simulink model "EKFSim_R2016b"  (R2018b)
settings: Solver=VariableStepAuto  StartTime=0.0  StopTime=22500  RelTol=1e-3
undefined symbols (not defined in the file): sigbuilder_block
libraries: fl_lib x7, nesl_utility x7
settings Model: Creator=WL  LastModifiedBy=Alter
settings SFSimCC: SimUseLocalCustomCode=off
settings RTWCC: RTWUseLocalCustomCode=off
settings CodeAppCC: StateflowObjectComments=on

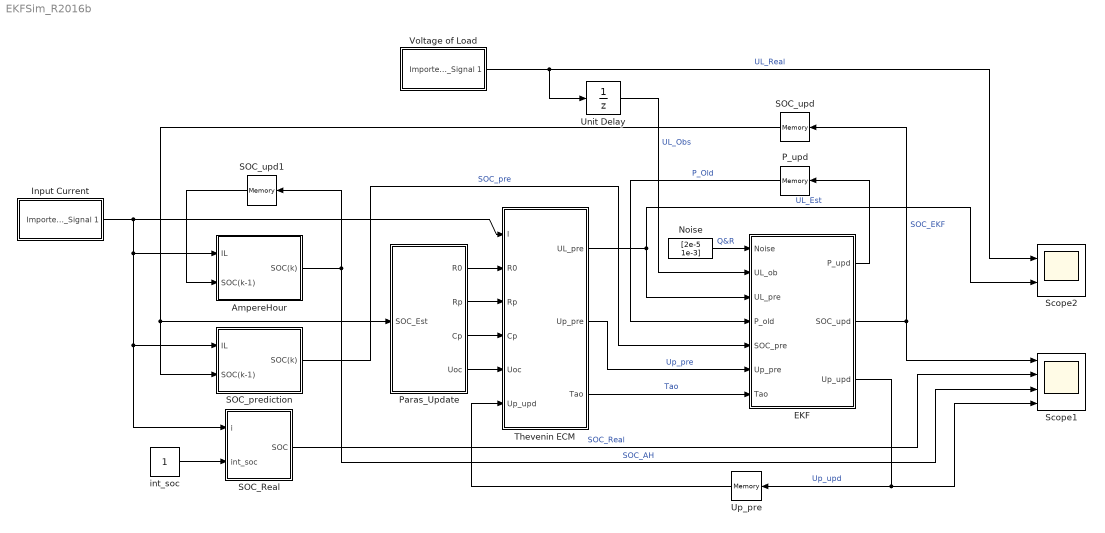
== system EKFSim_R2016b ==
  AmpereHour : Subsystem
  EKF : MATLAB Function  TreatAsAtomicUnit=on
  Input Current : Subsystem  Tag=STV Subsys  LoadFcn=sigbuilder_block('load');  StartFcn=sigbuilder_block('start');  StopFcn=sigbuilder_block('stop');  ClipboardFcn=sigbuilder_block('clipboard');  mask(Sigbuilder block){tuvar=[0:10]}
      mask help: Simulink:masks:SigbuilderBlock_MD
      mask init:
      | if ~strcmp(get_param(bdroot(gcbh),'SimulationStatus'),'stopped') tuvar = sigbuilder_block('maskInit'); end
      settings: CopyFcn=sigbuilder_block('copy');  DeleteFcn=sigbuilder_block('delete');  ModelCloseFcn=sigbuilder_block('modelClose');  PreSaveFcn=sigbuilder_block('preSave');  PauseFcn=sigbuilder_block('pause');  ContinueFcn=sigbuilder_block('continue');  NameChangeFcn=sigbuilder_block('namechange');  OpenFcn=sigbuilder_block('open',[6 51 1012.5 460.5 ]);  CloseFcn=sigbuilder_block('close');
      mask Display: plot(0, 0, 100, 100,[2, 2, 32, 32, 2], [68, 8, 8, 68, 68],[32, 2], [38, 38], [32, 19, 2],[53, 60, 44], [32, 17, 17, 2],[16, 16, 31, 31]);txt = getActiveGroup(gcbh);text(2, 100, txt,'verticalAlignment', 'top');
  Noise : Constant  Value=[2e-5 1e-3]
  P_upd : Memory  InitialCondition=[0.02 0 0 0.01]  InheritSampleTime=on  LinearizeAsDelay=on
  Paras_Update : Subsystem
  SOC_Real : Subsystem
  SOC_prediction : Subsystem
  SOC_upd : Memory  InitialCondition=1  InheritSampleTime=on  LinearizeAsDelay=on
  SOC_upd1 : Memory  InitialCondition=1  InheritSampleTime=on  LinearizeAsDelay=on
  Scope1 : Scope  NumInputPorts=4
  Scope2 : Scope  NumInputPorts=2
  Thevenin ECM : Subsystem
  Unit Delay : UnitDelay  InitialCondition=4.107  SampleTime=0.1
  Up_pre : Memory  InheritSampleTime=on  LinearizeAsDelay=on
  Voltage of Load : Subsystem  Tag=STV Subsys  LoadFcn=sigbuilder_block('load');  StartFcn=sigbuilder_block('start');  StopFcn=sigbuilder_block('stop');  ClipboardFcn=sigbuilder_block('clipboard');  mask(Sigbuilder block){tuvar=[0:10]}
      mask help: Simulink:masks:SigbuilderBlock_MD
      mask init:
      | if ~strcmp(get_param(bdroot(gcbh),'SimulationStatus'),'stopped') tuvar = sigbuilder_block('maskInit'); end
      settings: CopyFcn=sigbuilder_block('copy');  DeleteFcn=sigbuilder_block('delete');  ModelCloseFcn=sigbuilder_block('modelClose');  PreSaveFcn=sigbuilder_block('preSave');  PauseFcn=sigbuilder_block('pause');  ContinueFcn=sigbuilder_block('continue');  NameChangeFcn=sigbuilder_block('namechange');  OpenFcn=sigbuilder_block('open',[6 51 1012.5 460.5 ]);  CloseFcn=sigbuilder_block('close');
      mask Display: plot(0, 0, 100, 100,[2, 2, 32, 32, 2], [68, 8, 8, 68, 68],[32, 2], [38, 38], [32, 19, 2],[53, 60, 44], [32, 17, 17, 2],[16, 16, 31, 31]);txt = getActiveGroup(gcbh);text(2, 100, txt,'verticalAlignment', 'top');
  int_soc : Constant
  wires:
  Paras_Update/4(Uoc) -> Thevenin ECM/5(Uoc)
  Paras_Update/1(R0) -> Thevenin ECM/2(R0)
  int_soc/1 -> SOC_Real/2(int_soc)
  Paras_Update/3(Cp) -> Thevenin ECM/4(Cp)
  Paras_Update/2(Rp) -> Thevenin ECM/3(Rp)
  Thevenin ECM/1(UL_pre) -> Scope2/2, EKF/3(UL_pre)  "UL_Est"
  Voltage of Load/1(Imported_Signal 1) -> Unit Delay/1, Scope2/1  "UL_Real"
  SOC_Real/1(SOC) -> Scope1/2  "SOC_Real"
  Thevenin ECM/2(Up_pre) -> EKF/6(Up_pre)  "Up_pre"
  Noise/1 -> EKF/1(Noise)  "Q&R"
  SOC_prediction/1(SOC(k)) -> EKF/5(SOC_pre)  "SOC_pre"
  P_upd/1 -> EKF/4(P_old)  "P_Old"
  SOC_upd/1 -> SOC_prediction/2(SOC(k-1)), Paras_Update/1(SOC_Est)
  EKF/1(P_upd) -> P_upd/1
  Thevenin ECM/3(Tao) -> EKF/7(Tao)  "Tao"
  EKF/3(Up_upd) -> Scope1/4, Up_pre/1  "Up_upd"
  Up_pre/1 -> Thevenin ECM/6(Up_upd)
  EKF/2(SOC_upd) -> Scope1/1, SOC_upd/1  "SOC_EKF"
  Unit Delay/1 -> EKF/2(UL_ob)  "UL_Obs"
  AmpereHour/1(SOC(k)) -> Scope1/3, SOC_upd1/1  "SOC_AH"
  Input Current/1(Imported_Signal 1) -> SOC_prediction/1(IL), SOC_Real/1(i), AmpereHour/1(IL), Thevenin ECM/1(I)
  SOC_upd1/1 -> AmpereHour/2(SOC(k-1))

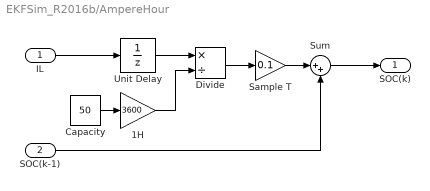
== system EKFSim_R2016b/AmpereHour ==
  IL : Inport
  SOC(k-1) : Inport  Port=2
  1H : Gain  Gain=3600
  Capacity : Constant  Value=50
  Divide : Product  Inputs=*/
  Sample T : Gain  Gain=0.1
  Sum : Sum  Inputs=|++
  Unit Delay : UnitDelay  SampleTime=0.15
  SOC(k) : Outport
  wires:
  Sample T/1 -> Sum/1
  Unit Delay/1 -> Divide/1
  SOC(k-1)/1 -> Sum/2
  IL/1 -> Unit Delay/1
  Sum/1 -> SOC(k)/1
  Capacity/1 -> 1H/1
  1H/1 -> Divide/2
  Divide/1 -> Sample T/1

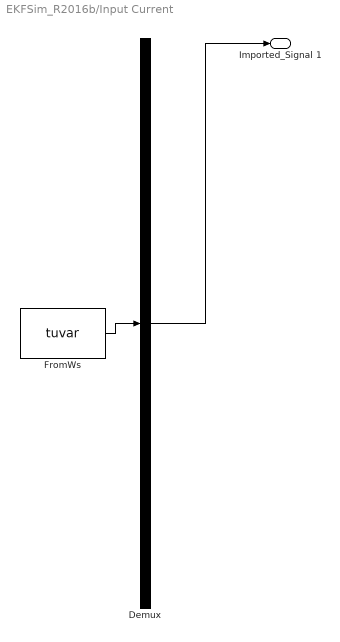
== system EKFSim_R2016b/Input Current ==
  Demux : Demux  Tag=STV Demux  Outputs=1
  FromWs : FromWorkspace  Tag=STV FromWs  VariableName=tuvar  SampleTime=0
      SigBuilderData=|
      | common.afterFinalStr = 'Extrapolate'
      | common.sampleTime = 0
      | dataSet.timeRange = [0 22502.2]
      | dataSet.name = 'I'
      | sbobj.Name = 'Signal Builder'
      | sbobj.Groups.Name = 'I'
      | sbobj.Groups.Signals.Name = 'Imported_Signal 1'
      | sbobj.Groups.Signals.XData = [0 0.05 0.1 0.15 0.2 0.25 0.3 0.35 0.4 0.45 0.5 0.55 ... (450045 elements, 1x450045)]
      | sbobj.Groups.Signals.YData = [0 0 0 0 0 0 0 0 0 0 0 0 ... (450045 elements, 1x450045)]
      | sbobj.Groups.TimeRange = [433.3 22935.5]
  Imported_Signal 1 : Outport
  wires:
  Demux/1 -> Imported_Signal 1/1
  FromWs/1 -> Demux/1

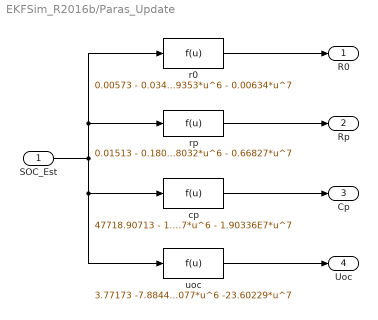
== system EKFSim_R2016b/Paras_Update ==
  SOC_Est : Inport
  cp : Fcn  Expr=47718.90713 - 1.00583E6*u^1 + 9.2653E6*u^2 - 3.91088E7*u^3 + 8.85892E7*u^4 - 1.11014E8*u^5 + 7.22811E7*u^6 - 1.90336E7*u^7
  r0 : Fcn  Expr=0.00573 - 0.03427*u^1 + 0.1455*u^2 - 0.32647*u^3 + 0.41465*u^4 - 0.28992*u^5 + 0.09353*u^6 - 0.00634*u^7
  rp : Fcn  Expr=0.01513 - 0.18008*u^1 + 1.05147*u^2 - 3.27616*u^3 + 5.79793*u^4 - 5.81819*u^5 + 3.08032*u^6 - 0.66827*u^7
  uoc : Fcn  Expr=3.77173 -7.88447*u^1 + 60.21383*u^2 -200.15462*u^3 + 345.34531*u^4 - 314.92282*u^5 + 141.34077*u^6 -23.60229*u^7
  R0 : Outport
  Rp : Outport  Port=2
  Cp : Outport  Port=3
  Uoc : Outport  Port=4
  wires:
  cp/1 -> Cp/1
  rp/1 -> Rp/1
  uoc/1 -> Uoc/1
  r0/1 -> R0/1
  SOC_Est/1 -> uoc/1, cp/1, rp/1, r0/1

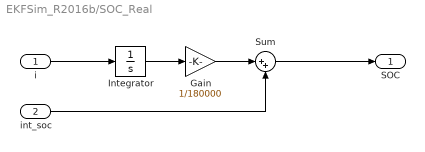
== system EKFSim_R2016b/SOC_Real ==
  i : Inport
  int_soc : Inport  Port=2
  Gain : Gain  Gain=1/180000
  Integrator : Integrator
  Sum : Sum  Inputs=|++
  SOC : Outport
  wires:
  Gain/1 -> Sum/1
  Integrator/1 -> Gain/1
  int_soc/1 -> Sum/2
  i/1 -> Integrator/1
  Sum/1 -> SOC/1

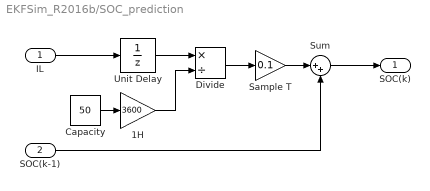
== system EKFSim_R2016b/SOC_prediction ==
  IL : Inport
  SOC(k-1) : Inport  Port=2
  1H : Gain  Gain=3600
  Capacity : Constant  Value=50
  Divide : Product  Inputs=*/
  Sample T : Gain  Gain=0.1
  Sum : Sum  Inputs=|++
  Unit Delay : UnitDelay  SampleTime=0.15
  SOC(k) : Outport
  wires:
  Sample T/1 -> Sum/1
  Unit Delay/1 -> Divide/1
  SOC(k-1)/1 -> Sum/2
  IL/1 -> Unit Delay/1
  Sum/1 -> SOC(k)/1
  Capacity/1 -> 1H/1
  1H/1 -> Divide/2
  Divide/1 -> Sample T/1

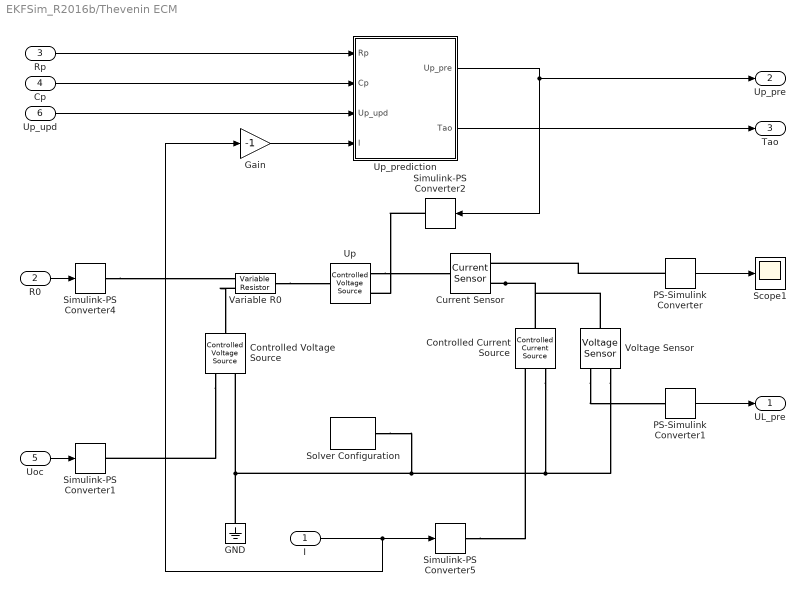
== system EKFSim_R2016b/Thevenin ECM ==
  I : Inport
  R0 : Inport  Port=2
  Rp : Inport  Port=3
  Cp : Inport  Port=4
  Uoc : Inport  Port=5
  Up_upd : Inport  Port=6
  Controlled Current Source : fl_lib/Electrical/Electrical Sources/Controlled Current Source
  Controlled Voltage Source : fl_lib/Electrical/Electrical Sources/Controlled Voltage Source
  Current Sensor : fl_lib/Electrical/Electrical Sensors/Current Sensor
  GND : fl_lib/Electrical/Electrical Elements/Electrical Reference
  Gain : Gain  Gain=-1
  PS-Simulink Converter : nesl_utility/PS-Simulink Converter  PhysicalDomain=network_engine_domain  SubClassName=ps_output  LeftPortType=input  RightPortType=output  PseudoPeriodic=off  Frequencies=[]  Unit=A  AffineConversion=off
  PS-Simulink Converter1 : nesl_utility/PS-Simulink Converter  PhysicalDomain=network_engine_domain  SubClassName=ps_output  LeftPortType=input  RightPortType=output  PseudoPeriodic=off  Frequencies=[]  Unit=V  AffineConversion=off
  Scope1 : Scope
  Simulink-PS Converter{1..2,4..5} (4 alike) : nesl_utility/Simulink-PS Converter  PhysicalDomain=network_engine_domain  SubClassName=ps_input  LeftPortType=input  RightPortType=output  PseudoPeriodic=off  Frequencies=[]  NoiseDistribution=none  NoiseParameters=[]  Unit=1  AffineConversion=off  FilteringAndDerivatives=zero  SimscapeFilterOrder=1  InputFilterTimeConstant=0.001  UdotUserProvided=0
  Solver Configuration : nesl_utility/Solver Configuration  PhysicalDomain=network_engine_domain  SubClassName=solver  LeftPortType=input  RightPortType=generic  Tones=[]  Harmonics=[]  SimulateNoise=off  Profile=off  UseLocalSampling=off  EnableSwitchedLinearOptims=on  FrequencyDomain=off  UseCCode=off  RelTol=0.001  AbsTol=1e-06  MinStep=1e-09  ToWorkspace=off  RevertToSquareIcSolve=off  NumHomotopyIterations=100  PhasorMode=off  PhasorModeNumHarmonics=1  DoDC=off  ResidualTolerance=1e-09  UseLocalSolver=off  LocalSolverChoice=NE_BACKWARD_EULER_ADVANCER  LocalSolverSampleTime=0.001  DoFixedCost=off  MaxNonlinIter=3  MaxModeIter=2  LinearAlgebra=Sparse  EquationFormulation=NE_TIME_EF  DelaysMemoryBudget=1024  AutomaticFiltering=on  FilteringTimeConstant=0.001  PartitionStorageMethod=AS_NEEDED  PartitionMemoryBudget=1024
  Up : fl_lib/Electrical/Electrical Sources/Controlled Voltage Source
  Up_prediction : MATLAB Function  TreatAsAtomicUnit=on
  Variable R0 : fl_lib/Electrical/Electrical Elements/Variable Resistor  Rmin=0 Ohm  i_specify=off  i_priority=None  i=0 A  i_nominal_specify=off  i_nominal_unit=A  i_nominal_value=1  v_specify=off  v_priority=None  v=0 V  v_nominal_specify=off  v_nominal_unit=V  v_nominal_value=1
  Voltage Sensor : fl_lib/Electrical/Electrical Sensors/Voltage Sensor
  UL_pre : Outport
  Up_pre : Outport  Port=2
  Tao : Outport  Port=3
  wires:
  PS-Simulink Converter1/1 -> UL_pre/1
  Uoc/1 -> Simulink-PS Converter1/1
  Cp/1 -> Up_prediction/2(Cp)
  Rp/1 -> Up_prediction/1(Rp)
  R0/1 -> Simulink-PS Converter4/1
  I/1 -> Gain/1, Simulink-PS Converter5/1
  PS-Simulink Converter/1 -> Scope1/1
  Up_prediction/1(Up_pre) -> Simulink-PS Converter2/1, Up_pre/1
  Up_upd/1 -> Up_prediction/3(Up_upd)
  Up_prediction/2(Tao) -> Tao/1
  Gain/1 -> Up_prediction/4(I)
  connections:
  Variable R0/LConn2 -- Controlled Voltage Source/LConn1
  Current Sensor/RConn2 -- Voltage Sensor/LConn1 -- Controlled Current Source/LConn1
  Voltage Sensor/RConn2 -- Controlled Current Source/RConn2 -- Solver Configuration/RConn1 -- Controlled Voltage Source/RConn2 -- GND/LConn1
  PS-Simulink Converter/LConn1 -- Current Sensor/RConn1
  Voltage Sensor/RConn1 -- PS-Simulink Converter1/LConn1
  Controlled Voltage Source/RConn1 -- Simulink-PS Converter1/RConn1
  Simulink-PS Converter5/RConn1 -- Controlled Current Source/RConn1
  Simulink-PS Converter4/RConn1 -- Variable R0/LConn1
  Variable R0/RConn1 -- Up/LConn1
  Up/RConn2 -- Current Sensor/LConn1
  Simulink-PS Converter2/RConn1 -- Up/RConn1

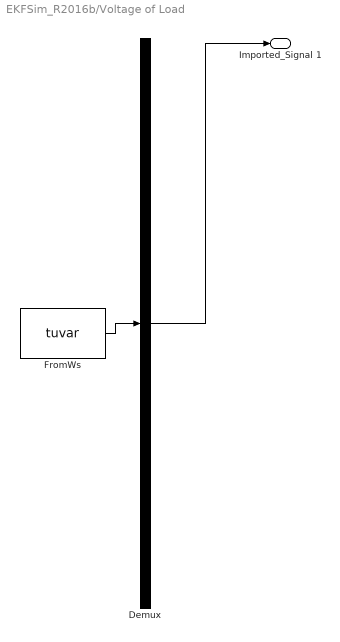
== system EKFSim_R2016b/Voltage of Load ==
  Demux : Demux  Tag=STV Demux  Outputs=1
  FromWs : FromWorkspace  Tag=STV FromWs  VariableName=tuvar  SampleTime=0
      SigBuilderData=|
      | common.afterFinalStr = 'Extrapolate'
      | common.sampleTime = 0
      | dataSet.timeRange = [0 22502.2]
      | dataSet.name = 'U'
      | sbobj.Name = 'Signal Builder'
      | sbobj.Groups.Name = 'U'
      | sbobj.Groups.Signals.Name = 'Imported_Signal 1'
      | sbobj.Groups.Signals.XData = [0 0.05 0.1 0.15 0.2 0.25 0.3 0.35 0.4 0.45 0.5 0.55 ... (450045 elements, 1x450045)]
      | sbobj.Groups.Signals.YData = [4.108 4.10766666667 4.10766666667 4.10766666667 4.10766666667 4.10766666667 4.10766666667 4.10766666667 4.10766666667 4.10766666667 4.10766666667 4.10833333333 ... (450045 elements, 1x450045)]
      | sbobj.Groups.TimeRange = [0 22502.2]
  Imported_Signal 1 : Outport
  wires:
  Demux/1 -> Imported_Signal 1/1
  FromWs/1 -> Demux/1

== matlab function EKFSim_R2016b/Thevenin ECM/Up_prediction ==
  data: Rp input; Up_pre output; Cp input; Up_upd input; Tao output; I input
function [Up_pre, Tao] = fcn(Rp, Cp,Up_upd,I)
Tao = Rp*Cp;
Up_pre=exp(-0.1/Tao)*Up_upd+Rp*(1-exp(-0.1/Tao))*I;

== matlab function EKFSim_R2016b/EKF ==
  data: P_upd output; Noise input; UL_ob input; UL_pre input; P_old input; SOC_pre input; Up_pre input; Tao input; SOC_upd output; Up_upd output
function [P_upd,SOC_upd,Up_upd] = EKF(Noise, UL_ob, UL_pre, P_old, SOC_pre, Up_pre, Tao)
Q = Noise(1);   %过程噪声
R = Noise(2);   %观测噪声

% --------------A矩阵，状态转移----------
A1 = 1;
A2 = exp(-0.05/Tao);
A = [A1 0;0 A2];

P_last = [P_old(1) P_old(2);P_old(3) P_old(4)];
P_pre=A*P_last*A'+ [Q 0;0 Q];  
%% --------------C矩阵-------------
C1 = -7.88447 + 60.21383*2*SOC_pre - 200.15462*3*SOC_pre^2 ...
    + 345.34531*4*SOC_pre^3 - 314.92282*5*SOC_pre^4 ...
    + 141.34077*6*SOC_pre^5 - 23.60229*5*SOC_pre^6;
C = [C1 -1];
%% --------------更新--------------
X_pre = [SOC_pre;Up_pre];
K = P_pre*C'*(C*P_pre*C'+ R)^(-1);     %增益
X_upd = X_pre + K*(UL_ob-UL_pre);     %得到估计值
P_update = P_pre - K*C*P_pre;
%% --------------输出--------------
SOC_upd = X_upd(1);
Up_upd = X_upd(2);
P_upd = [P_update(1,1) P_update(1,2) P_update(2,1) P_update(2,2)];
